simulink library "combinedHighLowFreqDataPlanarWave"  (R2020a)
settings: Solver=VariableStepAuto  StartTime=0.0  StopTime=10.0  RelTol=1e-3
libraries: lowFreqWithFAUTurb_cl x1, planarWaveModel_ul x1, constXYZT_PlanarWave_cl x1
settings Model: Creator=jcreed2  LastModifiedBy=jcreed2

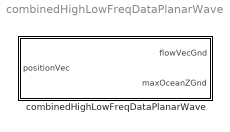
== system combinedHighLowFreqDataPlanarWave ==
  combinedHighLowFreqDataPlanarWave : Subsystem

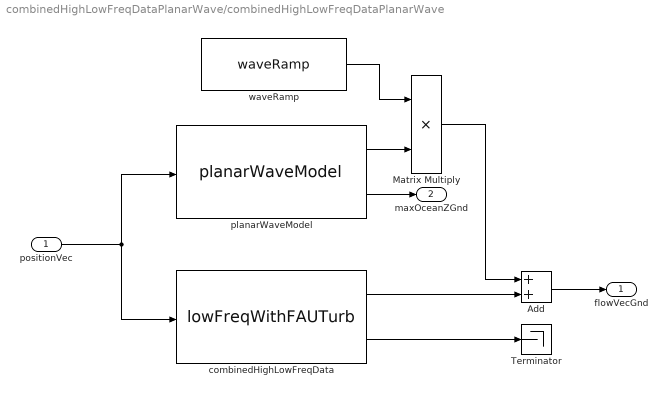
== system combinedHighLowFreqDataPlanarWave/combinedHighLowFreqDataPlanarWave ==
  positionVec : Inport
  Add : Sum
  Matrix Multiply : Product
  Terminator : Terminator
  combinedHighLowFreqData : lowFreqWithFAUTurb_cl/lowFreqWithFAUTurb  SystemSampleTime=-1  VariantControl=VSS_flowCalculation_combinedHighLowFreqData  Latency=0  AutoFrameSizeCalculation=off
  planarWaveModel : planarWaveModel_ul/planarWaveModel  SystemSampleTime=-1  Latency=0  AutoFrameSizeCalculation=off
  waveRamp : constXYZT_PlanarWave_cl/constXYZT_PlanarWave/waveRamp  SystemSampleTime=-1  Latency=0  AutoFrameSizeCalculation=off
  flowVecGnd : Outport  VectorParamsAs1DForOutWhenUnconnected=off
  maxOceanZGnd : Outport  Port=2  VectorParamsAs1DForOutWhenUnconnected=off
  wires:
  Add/1 -> flowVecGnd/1
  Matrix Multiply/1 -> Add/1
  planarWaveModel/1 -> Matrix Multiply/2
  positionVec/1 -> combinedHighLowFreqData/1, planarWaveModel/1
  combinedHighLowFreqData/2 -> Terminator/1
  planarWaveModel/2 -> maxOceanZGnd/1
  waveRamp/1 -> Matrix Multiply/1
  combinedHighLowFreqData/1 -> Add/2
